simulink model "lb332_sdruFreqCalibRx1"  (R2018b)
settings: Solver=VariableStepAuto  StartTime=0.0  StopTime=inf  RelTol=1e-3
PreLoadFcn:
  | Fs = 200e3; % Частота дискретизации, выборок в с
  | 
  | % Инициализация параметров приема устройства USRP
  | rxradio.MasterClockRate   = 20e6;   % тактовая частота, Гц
  | rxradio.CenterFrequency   = 450e6; % центральная частота
  | rxradio.Gain                    = 40;       % усиление, дБ
  | % Коэффициент децимации
  | rxradio.DecimationFactor  = rxradio.MasterClockRate/Fs;
  | rxradio.SamplesPerFrame  = 4096;  % выборок в кадре
libraries: commsdrhw_v2 x1
settings Model: Creator=Григорий Фокин  LastModifiedBy=Григорий Фокин

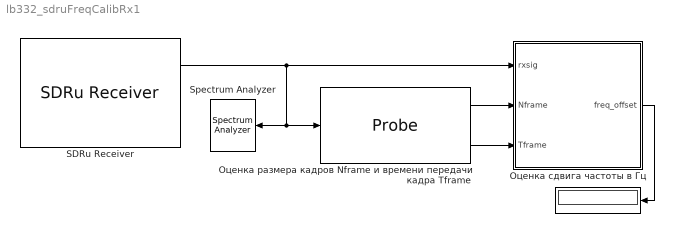
== system lb332_sdruFreqCalibRx1 ==
  " " : Display
  SDRu Receiver : commsdrhw_v2/SDRu Receiver  rxtx=rx  initializeIPAddress=0  devMap=0  USRP2_IP=192.168.10.2  USRP_IP_X300=192.168.10.2  USRP_IP_X310=192.168.10.2  USRP_serialNumB200=No devices found  USRP_serialNumB210=F4E642  platform=B210  prevPlatform=B210  lastIPAddressPopup=192.168.10.2  USRP_ID=F4E642  LastIPAddress=192.168.10.2  ChannelMapping=1  centerFrequencySrc=Dialog  centerFrequency=rxradio.CenterFrequency  loOffsetSrc=Dialog  loOffset=0  gainSrc=Dialog  gain=rxradio.Gain  PPSSource=Internal  clockSource=Internal  masterClkRateParam=20000000  masterClkRateB200=32e6  masterClkRateB210=rxradio.MasterClockRate  masterClkRateX300=200e6  masterClkRateX310=200e6  masterClkRate=100e6  decimInterpSrc=Dialog  decimInterp=rxradio.DecimationFactor  USRP2_IP_NUM=[70 52 69 54 52 50]  TransportDataType=int16  overrunUnderrunPort=off  sampleTime=1/Fs  outputDatatype=Same as transport data type  frameLength=rxradio.SamplesPerFrame  HOST_DATA_PORT=0  HOST_CONTROL_PORT=0  USRP2_DATA_PORT=0  USRP2_CONTROL_PORT=0  bufferMode=Continuous streaming  EnableBurstMode=off  NumFramesInBurst=100
      settings: SourceProductName=Communications System Toolbox Support Package for USRP(R) Radio  SourceProductBaseCode=USRP
  Spectrum Analyzer : SpectrumAnalyzer
  Оценка размера кадров Nframe и времени передачи кадра Tframe : Probe  ProbeComplexSignal=off
  Оценка сдвига частоты в Гц : MATLAB Function  TreatAsAtomicUnit=on
  wires:
  SDRu Receiver/1 -> Spectrum Analyzer/1, Оценка размера кадров Nframe и времени передачи кадра Tframe/1, Оценка сдвига частоты в Гц/1(rxsig)
  Оценка размера кадров Nframe и времени передачи кадра Tframe/2 -> Оценка сдвига частоты в Гц/3(Tframe)
  Оценка размера кадров Nframe и времени передачи кадра Tframe/1 -> Оценка сдвига частоты в Гц/2(Nframe)
  Оценка сдвига частоты в Гц/1(freq_offset) -> " "/1

== matlab function lb332_sdruFreqCalibRx1/Оценка сдвига частоты в Гц ==
  data: rxsig input; freq_offset output; Nframe input; Tframe input
function freq_offset  = freqoffset(rxsig, Nframe, Tframe)
% freq_offset - сдвиг частот, Гц
% rxsig - входной сигнал
% Nframe - число выборок в принимаемом кадре
% Tframe - время передачи кадра
Ts = Tframe(1)/Nframe;  % время дискретизации
Fs = 1/Ts;              % частота дискретизации входного сигнала, Гц
nfft = 2048;    % размерность БПФ
delta_f = Fs/nfft; % БПФ разрешение по частоте // fft bin
% Вычисление БПФ сигнала rxsig: [+ve freqs , -ve freqs]
fft_sig = fft(rxsig,nfft);    
% Преобразование сигнала fft_sig: [-ve freqs , +ve freqs]
fft_sig = fftshift(fft_sig);
% Нахождение индекса максимальной выборки fft_sig
[~, max_idx] = max(fft_sig); 
% Оценка индекса сдвига частот по индексу max_idx: 
% преобразование max_idx для симметрии относительно 0
offset_idx = max_idx-1-nfft/2;   
% Отображение индекса сдвига частот в значение сдвига частот
freq_offset = offset_idx*delta_f; 
end
